simulink model "AsyncIP_sl"  (R2021b)
settings: Solver=ode4  StartTime=0.0  StopTime=inf  FixedStep=.01  MaxStep=0.01  RelTol=1e-3  AbsTol=1e-6
InitFcn:
  | Ns=20;
undefined symbols (not defined in the file): IP, UDP
libraries: opal_lib x6, rtlab x3, rtio_generic_ip x1
settings Model: Creator=jwu  LastModifiedBy=NCSLab
settings SolverCC: AutoScaleAbsTol=off  AlgebraicLoopSolver=TrustRegion
settings DataIOCC: ExternalInput=[]  InitialState=[]  SaveFormat=Array  SignalLoggingSaveFormat=ModelDataLogs  SaveOutput=off  SaveTime=off  ReturnWorkspaceOutputs=off  SignalLoggingName=sigsOut
settings OptimizationCC: BooleanDataType=off  OptimizeBlockIOStorage=off  BufferReuse=off  ExpressionFolding=off  LocalBlockOutputs=off  InitFltsAndDblsToZero=on  LifeSpan=inf
settings DebuggingCC: SaveWithParameterizedLinksMsg=none  UnderspecifiedInitializationDetection=Classic  MergeDetectMultiDrivingBlocksExec=none  SignalResolutionControl=TryResolveAllWithWarning  InheritedTsInSrcMsg=none  MultiTaskDSMMsg=warning  MultiTaskCondExecSysMsg=none  FcnCallInpInsideContextMsg=warning  SFUnexpectedBacktrackingDiag=warning  SFNoUnconditionalDefaultTransitionDiag=warning  SFExecutionAtInitializationDiag=none  SFMachineParentedDataDiag=warning  ArithmeticOperatorsInVariantConditions=warning
settings HardwareCC: ProdBitPerPointer=32  ProdBitPerSizeT=32  ProdBitPerPtrDiffT=32  ProdLargestAtomicFloat=None  ProdIntDivRoundTo=Undefined  ProdEndianess=Unspecified  ProdWordSize=32  ProdHWDeviceType=32-bit Generic  TargetUnknown=on
settings ModelReferenceCC: PropagateSignalLabelsOutOfModel=off
settings SFSimCC: SimUseLocalCustomCode=off  CustomCodeUndefinedFunction=UseInterfaceOnly
settings RTWCC: RTWUseLocalCustomCode=off
settings CodeAppCC: StateflowObjectComments=on
settings GRTTargetCC: TargetFcnLib=ansi_tfl_tmw.mat  TargetLangStandard=C89/C90 (ANSI)  CombineOutputUpdateFcns=off  GRTInterface=on
settings ConfigComp: CovMetricSettings=dw  CovSaveCumulativeToWorkspaceVar=on  CovSaveSingleToWorkspaceVar=on  CovExternalEMLEnable=off

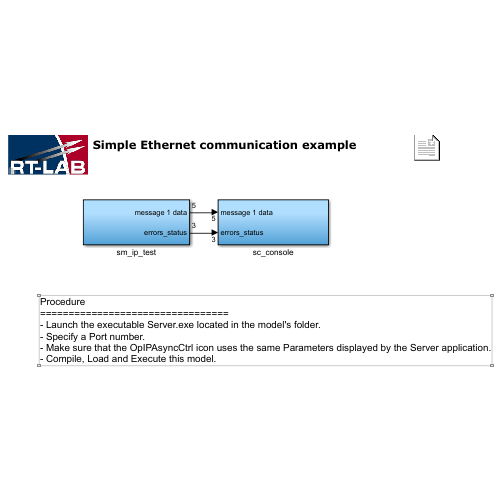
[thumbnail: Simulink's stored preview of the top-level diagram]
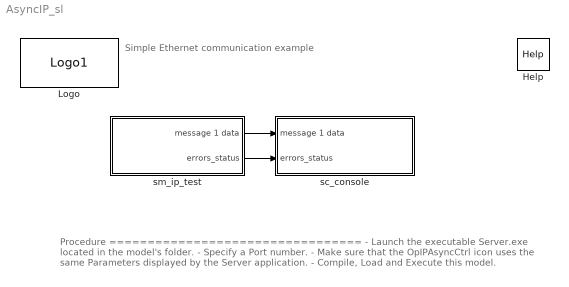
== system AsyncIP_sl ==
  note: Simple Ethernet communication example
  note: Procedure
      | =================================
      | - Launch the executable Server.exe located in the model's folder.
      | - Specify a Port number.
      | - Make sure that the OpIPAsyncCtrl icon uses the same Parameters displayed by the Server application.
      | - Compile, Load and Execute this model.
  Help : opal_lib/Help  docfile=../../help/help.simulink.html
  Logo : opal_lib/Logo1  vide=[]
  sc_console : Subsystem
  sm_ip_test : Subsystem
  wires:
  sm_ip_test/1(message 1 data) -> sc_console/1(message 1 data)
  sm_ip_test/2(errors_status) -> sc_console/2(errors_status)

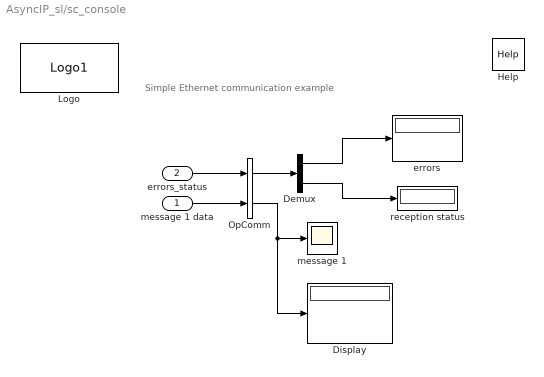
== system AsyncIP_sl/sc_console ==
  note: Simple Ethernet communication example
  message 1 data : Inport
  errors_status : Inport  Port=2
  Demux : Demux  Outputs=[2 1]
      settings: DisplayOption=none
  Display : Display
  Help : opal_lib/Help  docfile=../../help/help.simulink.html
  Logo : opal_lib/Logo1  vide=[]
  OpComm : rtlab/OpComm  nbport=2  groupe_acq=1  subsys_rate=0  st=0  Synchronization=on  Interpolation=on  Threshold=1.0  Missed_Data=off  Sim_Time=off  Samples=off  dynSigOut=off  from_console=0  warning_done=off  writeOpCommFile=off  Offset=off
      settings: SourceProductName=RT-LAB
  errors : Display
  message 1 : Scope
  reception status : Display
  wires:
  errors_status/1 -> OpComm/1
  OpComm/2 -> message 1/1, Display/1
  message 1 data/1 -> OpComm/2
  OpComm/1 -> Demux/1
  Demux/1 -> errors/1
  Demux/2 -> reception status/1

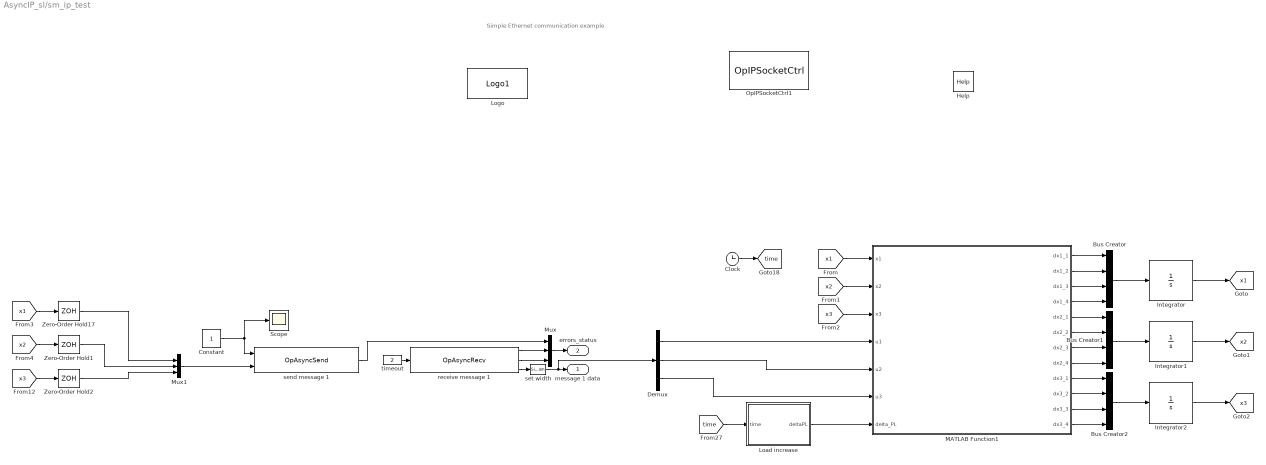
== system AsyncIP_sl/sm_ip_test ==
  note: Simple Ethernet communication example
  Bus Creator : BusCreator  Inputs=4
  Bus Creator1 : BusCreator  Inputs=4
  Bus Creator2 : BusCreator  Inputs=4
  Clock : Clock
  Constant : Constant
  Demux : Demux  Outputs=3
  Help : opal_lib/Help  docfile=../../help/help.simulink.html
  Integrator : Integrator  InitialCondition=zeros(4,1)
  Integrator1 : Integrator  InitialCondition=zeros(4,1)
  Integrator2 : Integrator  InitialCondition=zeros(4,1)
  Load increase : MATLAB Function  TreatAsAtomicUnit=on
  Logo : opal_lib/Logo1  vide=[]
  MATLAB Function1 : MATLAB Function  TreatAsAtomicUnit=on
  Mux : Mux  Inputs=3
  Mux1 : Mux  Inputs=3
  OpIPSocketCtrl1 : rtio_generic_ip/OpIPSocketCtrl  ctl_id=1  proto=UDP/IP  ip_addr_remote=10.64.117.70  ip_port_remote=8080  ip_port_local=8080  ip_addr_mcast=0.0.0.0  exe_name=AsyncIP
      settings: SourceProductName=RT-LAB I/O
  Scope : Scope
  Zero-Order Hold1 : ZeroOrderHold  SampleTime=Ns*5e-4
  Zero-Order Hold17 : ZeroOrderHold  SampleTime=Ns*5e-4
  Zero-Order Hold2 : ZeroOrderHold  SampleTime=Ns*5e-4
  receive message 1 : rtlab/Communication/Asynchronous/OpAsyncRecv  ctl_id=1  recv_id=1  enable_param=off  fp1=1  fp2=2  fp3=3  fp4=4  fp5=5  sp1=string1  sp2=string2  sp3=string3  sp4=string4  sp5=string5  fp6=6  fp7=7
      settings: SourceProductName=RT-LAB
  send message 1 : rtlab/Communication/Asynchronous/OpAsyncSend  ctl_id=1  send_id=1  mode=DONT_NEED_REPLY  enable_param=off  fp1=1  fp2=2  fp3=3  fp4=4  fp5=5  sp1=string1  sp2=string2  sp3=string3  sp4=string4  sp5=string5
      settings: SourceProductName=RT-LAB
  set width : SignalSpecification  Dimensions=3
  timeout : Constant  Value=2
  message 1 data : Outport
  errors_status : Outport  Port=2
  tag scope: time=global, x1=global, x2=global, x3=global
  wires:
  receive message 1/3 -> set width/1
  receive message 1/1 -> Mux/2
  receive message 1/2 -> Mux/3
  timeout/1 -> receive message 1/1
  Constant/1 -> send message 1/1, Scope/1
  send message 1/1 -> Mux/1
  Mux/1 -> errors_status/1
  set width/1 -> Demux/1, message 1 data/1
  Demux/1 -> MATLAB Function1/4(u1)
  [time] -> Load increase/1(time)
  Load increase/1(deltaPL) -> MATLAB Function1/7(delta_PL)
  MATLAB Function1/4(dx1_4) -> Bus Creator/4
  [x3] -> MATLAB Function1/3(x3)
  MATLAB Function1/1(dx1_1) -> Bus Creator/1
  Clock/1 -> [time]
  MATLAB Function1/9(dx3_1) -> Bus Creator2/1
  MATLAB Function1/7(dx2_3) -> Bus Creator1/3
  Demux/3 -> MATLAB Function1/6(u3)
  MATLAB Function1/11(dx3_3) -> Bus Creator2/3
  Integrator/1 -> [x1]
  MATLAB Function1/2(dx1_2) -> Bus Creator/2
  MATLAB Function1/12(dx3_4) -> Bus Creator2/4
  [x2] -> MATLAB Function1/2(x2)
  Integrator2/1 -> [x3]
  Bus Creator/1 -> Integrator/1
  Bus Creator2/1 -> Integrator2/1
  MATLAB Function1/6(dx2_2) -> Bus Creator1/2
  MATLAB Function1/5(dx2_1) -> Bus Creator1/1
  [x1] -> MATLAB Function1/1(x1)
  MATLAB Function1/10(dx3_2) -> Bus Creator2/2
  MATLAB Function1/8(dx2_4) -> Bus Creator1/4
  Bus Creator1/1 -> Integrator1/1
  MATLAB Function1/3(dx1_3) -> Bus Creator/3
  Integrator1/1 -> [x2]
  Demux/2 -> MATLAB Function1/5(u2)
  Zero-Order Hold17/1 -> Mux1/1
  [x1] -> Zero-Order Hold17/1
  [x2] -> Zero-Order Hold1/1
  Zero-Order Hold2/1 -> Mux1/3
  [x3] -> Zero-Order Hold2/1
  Zero-Order Hold1/1 -> Mux1/2
  Mux1/1 -> send message 1/2

== matlab function AsyncIP_sl/sm_ip_test/MATLAB Function1 ==
  data: x1 input; dx1_1 output; x2 input; x3 input; u1 input; u2 input; u3 input; dx1_2 output; dx1_3 output; dx1_4 output; dx2_1 output; dx2_2 output; dx2_3 output; dx2_4 output; dx3_1 output; dx3_2 output; dx3_3 output; dx3_4 output; delta_PL input
function [dx1_1,dx1_2,dx1_3,dx1_4,dx2_1,dx2_2,dx2_3,dx2_4,dx3_1,dx3_2,dx3_3,dx3_4] = fcn(x1,x2,x3,u1,u2,u3,delta_PL)
% function dx1 = fcn(x1,x2,x3,u1,u2,u3)
% x=zeros(3,4);
x=[x1';x2';x3'];
dx=zeros(3,4);
u=[u1;u2;u3];


M=1*[3.5 4 3.75];
D=1.1*[2 2.75 2.4];
% D=1.1*[2 2.75 3.4];
Tg=0.5*[40 25 32];
% Tg=1*[40 25 32];
Tch=1*[50 10 30];
Rw=1.5*[1 1 1];
% Rw=1*[1 1.2 2];
s=[0 0 0];
T=zeros(3,3);

T(1,2)=7.54;
T(1,3)=T(1,2);
T(2,1)=7.54;
T(2,3)=T(2,1);
T(3,1)=7.54;
T(3,2)=T(3,1);

w=zeros(2,3);
%%
% delta_PL=10*[0.2 0.2 0.2];
%%
delta_Pe=0*ones(1,3);
for i=1:3
    w(:,i)=[delta_PL(i); delta_Pe(i)];
end

bar_T=zeros(1,3);

for i=1:3
    for j=1:3
        bar_T(1,i)=bar_T(1,i)+T(i,j);
    end
end

A=cell(1,3);
A_=cell(3,3);
B=cell(1,3);
A_D=cell(1,3);

for i=1:3
    A{1,i}=[-D(i)/M(i) 1/M(i) 0 -1/M(i); 0 -1/Tch(i) 1/Tch(i) 0; -1/(Tg(i)*Rw(i)) 0 -1/Tg(i) 0; bar_T(i) 0 0 0];
    B{1,i}=[0; 0; 1/Tg(i); 0];
    A_D{1,i}=[-1/M(i) 0; 0 0; 0 s(i)/Tg(i); 0 0];
    for j=1:3
        A_{i,j}=-T(i,j)*[0 0 0 0; 0 0 0 0; 0 0 0 0; 1 0 0 0];
    end
end

%%
for i=1:3
    Inter=zeros(4,1);
    for j=1:3
        Inter=Inter+A_{i,j}*x(j,:)';
    end
    dx(i,:)=A{1,i}*x(i,:)'+Inter+B{1,i}*u(i)+A_D{1,i}*w(:,i);
end

%%
% dx(1,1:3)
dx1_1=dx(1,1);
dx1_2=dx(1,2);
dx1_3=dx(1,3);
dx1_4=dx(1,4);
% dx2=dx(2,:);
% dx3=dx(3,:);
dx2_1=dx(2,1);
dx2_2=dx(2,2);
dx2_3=dx(2,3);
dx2_4=dx(2,4);

dx3_1=dx(3,1);
dx3_2=dx(3,2);
dx3_3=dx(3,3);
dx3_4=dx(3,4);

== matlab function AsyncIP_sl/sm_ip_test/Load increase ==
  data: time input; deltaPL output
function deltaPL  = fcn(time)
deltaPL=zeros(1,3);
if time<5
    deltaPL=[0 0 0];
elseif time<10
    deltaPL=[2 0 0];
elseif time<15
    deltaPL=[2 2 0];
elseif time<20
    deltaPL=[2 2 2];
elseif time<200
    deltaPL=[2 2 3];
end
